simulink model "driveController"  (R2026a)
settings: Solver=FixedStepAuto  StopTime=20  FixedStep=0.001
StartFcn:
  | run("setupParams.m")
values from neighbouring files (symbols this model uses):
  aero_bal_r = 0.5    [setupParams.m]    (also in setupParamsSingle.m)
  Af = 1.1    [setupParams.m]    (also in setupParamsSingle.m)
  ay_limit = 15.0    (= 15)    [setupParams.m]    (also in setupParamsSingle.m)
  Cl = 1.0    (= 1)    [setupParams.m]    (also in setupParamsSingle.m)
  deathzone_APP = 5    [setupParams.m]    (also in setupParamsSingle.m)
  e_yaw_deadzone = 0.03    [setupParams.m]
  falling_slew_rate_torque = -500    [setupParams.m]    (also in setupParamsSingle.m)
  g = 9.81    [setupParams.m]    (also in setupParamsSingle.m)
  h_o = 0.35    [setupParams.m]    (also in setupParamsSingle.m)
  I_charge_max = 21    [setupParams.m]
  I_discharge_max = 90    [setupParams.m]
  K_roll_rear = 0.6    [setupParams.m]    (also in setupParamsSingle.m = 0.5)
  Kus = 0.03    [setupParams.m]    (also in setupParamsSingle.m = 0)
  l_f = 0.775    [setupParams.m]    (also in setupParamsSingle.m)
  launch_ramp_rate = 1000.0    (= 1000)    [setupParams.m]    (also in setupParamsSingle.m)
  launch_V_thresh = 5.0    (= 5)    [setupParams.m]    (also in setupParamsSingle.m)
  mass = 320    [setupParams.m]    (also in setupParamsSingle.m = 300)
  mu = 1.5    [setupParams.m]    (also in setupParamsSingle.m)
  nominal_ramp_rate = 1000.0    (= 1000)    [setupParams.m]    (also in setupParamsSingle.m)
  overslip_factor = 1.01    [setupParams.m]    (also in setupParamsSingle.m = 1.13)
  pedal_bp = (0:10:100)'    [setupParams.m]    (also in setupParamsSingle.m)
  pedal_map = (pedal_bp / 100) .^ pedal_alpha    [setupParams.m]    (also in setupParamsSingle.m = (pedal_bp / 100) .^ pedal_alpha.Value)
  R_wheel = 0.2032    [setupParams.m]    (also in setupParamsSingle.m)
  regen_I_cont_A = 14.0    (= 14)    [setupParams.m]    (also in setupParamsSingle.m)
  regen_I_peak_A = 21.0    (= 21)    [setupParams.m]    (also in setupParamsSingle.m)
  regen_I_peak_dur_s = 4.0    (= 4)    [setupParams.m]    (also in setupParamsSingle.m)
  regen_P_batt_max_W = 35000    [setupParams.m]    (also in setupParamsSingle.m)
  regen_pedal_thr = 5.0    (= 5)    [setupParams.m]    (also in setupParamsSingle.m = 10)
  regen_speed_crit_rpm = 1000    [setupParams.m]    (also in setupParamsSingle.m = 500)
  regen_speed_min_rpm = 4000    [setupParams.m]    (also in setupParamsSingle.m = 3000)
  regen_T_max = 9    [setupParams.m]    (also in setupParamsSingle.m = Simulink.Parameter(T_rated.Value/2))
  rho = 1.225    [setupParams.m]    (also in setupParamsSingle.m)
  rid_eff = 0.80    (= 0.8)    [setupParams.m]    (also in setupParamsSingle.m)
  rid_ratio = 15    [setupParams.m]    (also in setupParamsSingle.m)
  rising_slew_rate_torque = 100    [setupParams.m]    (also in setupParamsSingle.m)
  rpm_safe_threshold = 100    [setupParams.m]
  slip_bc_coeff = 10    [setupParams.m]    (also in setupParamsSingle.m = Simulink.Parameter(1.5))
  slip_filt_N = 80    [setupParams.m]    (also in setupParamsSingle.m = 15)
  slip_Kd = 0.8    [setupParams.m]    (also in setupParamsSingle.m = Simulink.Parameter(5.0))
  slip_Ki = 13.0    (= 13)    [setupParams.m]    (also in setupParamsSingle.m = Simulink.Parameter(110.0))
  slip_Kp = 50.0    (= 50)    [setupParams.m]    (also in setupParamsSingle.m = Simulink.Parameter(180.0))
  slip_low_sat = 0.0    (= 0)    [setupParams.m]    (also in setupParamsSingle.m)
  slip_up_sat = 25    [setupParams.m]    (also in setupParamsSingle.m = 21)
  slip_V_min = 3    [setupParams.m]    (also in setupParamsSingle.m = 1)
  steer_ratio = 4.2    [pure_pursuit.m]    (also in setupParams.m; setupParamsSingle.m)
  steering_deadband = 1    [setupParams.m]
  T_headroom_k = 13.0    (= 13)    [setupParams.m]    (also in setupParamsSingle.m = Simulink.Parameter(5.0))
  T_headroom_max = 9    [setupParams.m]    (also in setupParamsSingle.m = Simulink.Parameter(5.0))
  T_peak = 20    [setupParams.m]    (also in setupParamsSingle.m = 21)
  T_rated = 9.8    [setupParams.m]    (also in setupParamsSingle.m = Simulink.Parameter(9.8))
  track_width = (track_width_r + track_width_f)/2    (= 1.2)    [setupParams.m]    (also in setupParamsSingle.m = sqrt(track_width_r^2 + track_width_f^2))
  track_width_r = 1.2    [setupParams.m]    (also in setupParamsSingle.m)
  Ts = 0.01    [setupParams.m]    (also in setupParamsSingle.m)
  tvc_bc = 17    [setupParams.m]
  tvc_D_thresh = 0.060    (= 0.06)    [setupParams.m]    (also in setupParamsSingle.m)
  tvc_D_thresh_off = 0.03    [setupParams.m]    (also in setupParamsSingle.m)
  tvc_Kd = 100    [setupParams.m]    (also in setupParamsSingle.m = Simulink.Parameter(5))
  tvc_Ki = 150    [setupParams.m]    (also in setupParamsSingle.m = Simulink.Parameter(10))
  tvc_Kp = 650    [setupParams.m]    (also in setupParamsSingle.m = Simulink.Parameter(70))
  tvc_N_filter = 25    [setupParams.m]    (also in setupParamsSingle.m = Simulink.Parameter(20))
  tvc_sat_dMz = 700    [setupParams.m]    (also in setupParamsSingle.m = Simulink.Parameter(10.0))
  tvc_throttle_on = 3.0    (= 3)    [setupParams.m]    (also in setupParamsSingle.m = Simulink.Parameter(3.0))
  tvc_tr = 5    [setupParams.m]    (also in setupParamsSingle.m = Simulink.Parameter(1.0))
  tvc_V_off = 2.0    (= 2)    [setupParams.m]    (also in setupParamsSingle.m = Simulink.Parameter(2.0))
  tvc_V_on = 4.0    (= 4)    [setupParams.m]    (also in setupParamsSingle.m = Simulink.Parameter(4.0))
  tvc_yaw_thresh = 0.08    [setupParams.m]    (also in setupParamsSingle.m)
  tvc_yaw_thresh_off = 0.04    [setupParams.m]    (also in setupParamsSingle.m)
  V_dc = 540    [setupParams.m]    (also in setupParamsSingle.m)
  V_dc_p = Simulink.Parameter(V_dc)    [setupParams.m]
  wheelbase = l_f + l_r    (= 1.55)    [setupParams.m]    (also in setupParamsSingle.m)
libraries: simulink x5, slpidlib x3
settings Model: Creator=Utente  LastModifiedBy=Utente
settings SolverCC: EnableFixedStepZeroCrossing=on
settings HardwareCC: ProdLargestAtomicInteger=Long  ProdLargestAtomicFloat=Double  ProdHWDeviceType=ARM Compatible->ARM Cortex-M
settings RTWCC: SystemTargetFile=ert.tlc  GenCodeOnly=on  Toolchain=GNU Tools for STM32  DataTypeReplacement=CDataTypesFixedWidth  Description=Embedded Coder
settings ERTTargetCC: MaxIdInt64=INT64_MAX  MinIdInt64=INT64_MIN  MaxIdUint64=UINT64_MAX  MaxIdInt32=INT32_MAX  MinIdInt32=INT32_MIN  MaxIdUint32=UINT32_MAX  MaxIdInt16=INT16_MAX  MinIdInt16=INT16_MIN  MaxIdUint16=UINT16_MAX  MaxIdInt8=INT8_MAX  MinIdInt8=INT8_MIN  MaxIdUint8=UINT8_MAX  GenerateSampleERTMain=on

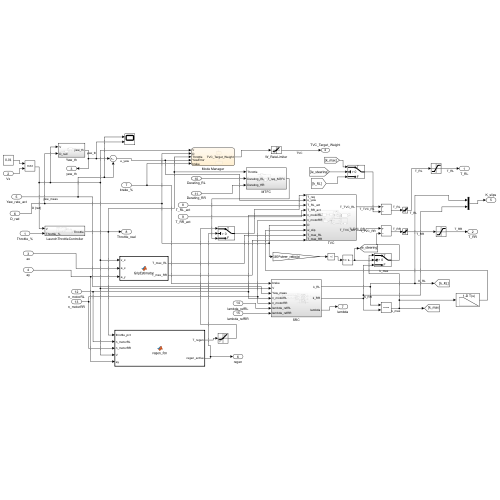
[thumbnail: Simulink's stored preview of the top-level diagram]
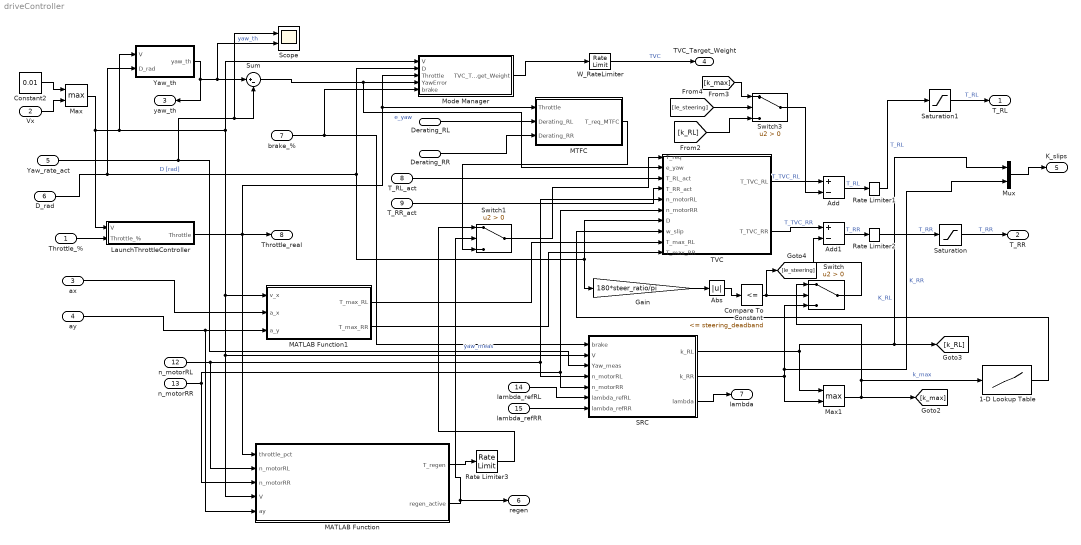
== system driveController ==
  Throttle_% : Inport
  Vx : Inport  Port=2
  ax : Inport  Port=3
  ay : Inport  Port=4
  Yaw_rate_act : Inport  Port=5
  D_rad : Inport  Port=6
  brake_% : Inport  Port=7
  T_RL_act : Inport  Port=8
  T_RR_act : Inport  Port=9
  Derating_RL : Inport  Port=10
  Derating_RR : Inport  Port=11
  n_motorRL : Inport  Port=12
  n_motorRR : Inport  Port=13
  lambda_refRL : Inport  Port=14
  lambda_refRR : Inport  Port=15
  1-D Lookup Table : Lookup_n-D  NumberOfTableDimensions=1  BreakpointsForDimension1=[0,3,12]  Table=[1,1,0]  ExtrapMethod=Clip  UseLastTableValue=on  InternalRulePriority=Speed  RndMeth=Simplest
  Abs : Abs  SaturateOnIntegerOverflow=off
  Add : Sum  Inputs=+-
  Add1 : Sum  Inputs=+-
  Compare To Constant : simulink/Logic and Bit Operations/Compare To Constant  relop=<=  const=steering_deadband  OutDataTypeStr=boolean
  Constant2 : Constant  Value=0.01
  Gain : Gain  Gain=180*steer_ratio/pi
  LaunchThrottleController : Subsystem
  MATLAB Function : MATLAB Function  TreatAsAtomicUnit=on
  MATLAB Function1 : MATLAB Function  TreatAsAtomicUnit=on
  MTFC : Subsystem
  Max : MinMax  Function=max  Inputs=2
  Max1 : MinMax  Function=max  Inputs=2
  Mode Manager : Stateflow chart  TreatAsAtomicUnit=on
  Mux : Mux  Inputs=2
  Rate Limiter1 : RateLimiter  RisingSlewLimit=rising_slew_rate_torque  FallingSlewLimit=falling_slew_rate_torque  SampleTimeMode=inherited
  Rate Limiter2 : RateLimiter  RisingSlewLimit=rising_slew_rate_torque  FallingSlewLimit=falling_slew_rate_torque  SampleTimeMode=inherited
  Rate Limiter3 : RateLimiter  RisingSlewLimit=60  FallingSlewLimit=-20  SampleTimeMode=inherited
  SRC : Subsystem
  Saturation : Saturate  UpperLimit=T_peak  LowerLimit=-regen_T_max
  Saturation1 : Saturate  UpperLimit=T_peak  LowerLimit=-regen_T_max
  Scope : Scope  NumInputPorts=2
      settings: ActiveDisplayYMinimum=-1.2846466868170756  ActiveDisplayYMaximum=1.5088492229704735
  Sum : Sum  Inputs=|+-
  Switch : Switch  Criteria=u2 > Threshold  SaturateOnIntegerOverflow=off  InputSameDT=off
  Switch1 : Switch  Criteria=u2 > Threshold  SaturateOnIntegerOverflow=off  InputSameDT=off
  Switch3 : Switch  Criteria=u2 > Threshold  SaturateOnIntegerOverflow=off  InputSameDT=off
  TVC : Subsystem
  W_RateLimiter : RateLimiter  RisingSlewLimit=2  FallingSlewLimit=-2  SampleTimeMode=inherited
  Yaw_th : Subsystem
  T_RL : Outport
  T_RR : Outport  Port=2
  yaw_th : Outport  Port=3
  TVC_Target_Weight : Outport  Port=4
  K_slips : Outport  Port=5
  regen : Outport  Port=6
  lambda : Outport  Port=7
  Throttle_real : Outport  Port=8
  wires:
  [k_RL] -> Switch3/3
  Add/1 -> Rate Limiter1/1  "T_RL"
  Mode Manager/1(TVC_Target_Weight) -> W_RateLimiter/1
  n_motorRR/1 -> TVC/6(n_motorRR), SRC/5(n_motorRR), MATLAB Function/3(n_motorRR)
  SRC/1(k_RL) -> Mux/1, [k_RL], Max1/1  "K_RL"
  Max1/1 -> 1-D Lookup Table/1, Switch/1, [k_max]  "k_max"
  [le_steering] -> Switch3/2
  Saturation/1 -> T_RR/1  "T_RR"
  n_motorRL/1 -> TVC/5(n_motorRL), SRC/4(n_motorRL), MATLAB Function/2(n_motorRL)
  T_RL_act/1 -> TVC/3(T_RL_act)
  T_RR_act/1 -> TVC/4(T_RR_act)
  MATLAB Function1/1(T_max_RL) -> TVC/9(T_max_RL)
  lambda_refRL/1 -> SRC/6(lambda_refRL)
  MATLAB Function/1(T_regen) -> Rate Limiter3/1
  ay/1 -> MATLAB Function/5(ay), MATLAB Function1/3(a_y)
  Yaw_rate_act/1 -> SRC/3(Yaw_meas), Scope/1, Sum/2  "yaw_meas"
  Constant2/1 -> Max/1
  Rate Limiter3/1 -> Switch1/1
  D_rad/1 -> TVC/7(D), Gain/1, Mode Manager/2(D), Yaw_th/2(D_rad)  "D [rad]"
  Derating_RR/1 -> MTFC/3(Derating_RR)
  Switch3/1 -> Add/2
  Add1/1 -> Rate Limiter2/1  "T_RR"
  Mux/1 -> K_slips/1
  brake_%/1 -> SRC/1(brake), Mode Manager/5(brake)
  W_RateLimiter/1 -> TVC_Target_Weight/1  "TVC"
  ax/1 -> MATLAB Function1/2(a_x)
  lambda_refRR/1 -> SRC/7(lambda_refRR)
  MATLAB Function1/2(T_max_RR) -> TVC/10(T_max_RR)
  Max/1 -> LaunchThrottleController/1(V), MATLAB Function/4(V), SRC/2(V), MATLAB Function1/1(v_x), Mode Manager/1(V), Yaw_th/1(V)
  LaunchThrottleController/1(Throttle) -> MATLAB Function/1(throttle_pct), Mode Manager/3(Throttle), MTFC/1(Throttle), Throttle_real/1
  Saturation1/1 -> T_RL/1  "T_RL"
  Vx/1 -> Max/2
  Yaw_th/1(yaw_th) -> Scope/2, Sum/1, yaw_th/1  "yaw_th"
  [k_max] -> Switch3/1
  MTFC/1(T_req_MTFC) -> Switch1/3
  TVC/1(T_TVC_RL) -> Add/1  "T_TVC_RL"
  Switch/1 -> Add1/2
  Compare To Constant/1 -> [le_steering], Switch/2
  MATLAB Function/2(regen_active) -> Switch1/2, regen/1
  1-D Lookup Table/1 -> TVC/8(w_slip)
  Switch1/1 -> TVC/1(T_req)
  TVC/2(T_TVC_RR) -> Add1/1  "T_TVC_RR"
  Derating_RL/1 -> MTFC/2(Derating_RL)
  Gain/1 -> Abs/1
  Throttle_%/1 -> LaunchThrottleController/2(Throttle_%)
  Abs/1 -> Compare To Constant/1
  Sum/1 -> TVC/2(e_yaw), Mode Manager/4(YawError)  "e_yaw"
  SRC/3(lambda) -> lambda/1
  Rate Limiter2/1 -> Saturation/1  "T_RR"
  Rate Limiter1/1 -> Saturation1/1  "T_RL"
  SRC/2(k_RR) -> Switch/3, Mux/2, Max1/2  "K_RR"

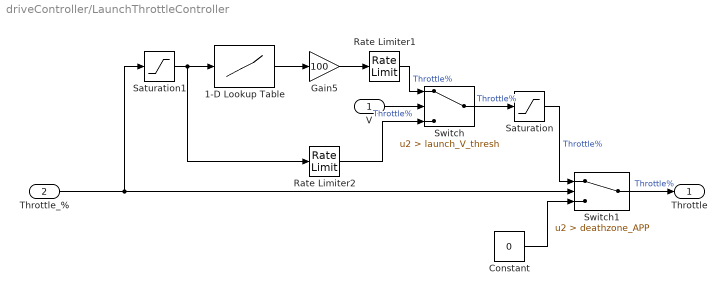
== system driveController/LaunchThrottleController ==
  V : Inport
  Throttle_% : Inport  Port=2
  1-D Lookup Table : Lookup_n-D  NumberOfTableDimensions=1  BreakpointsForDimension1=pedal_bp  Table=pedal_map  ExtrapMethod=Clip  UseLastTableValue=on  InternalRulePriority=Speed  RndMeth=Simplest
  Constant : Constant  Value=0
  Gain5 : Gain  Gain=100
  Rate Limiter1 : RateLimiter  RisingSlewLimit=launch_ramp_rate  FallingSlewLimit=-250  SampleTimeMode=inherited
  Rate Limiter2 : RateLimiter  RisingSlewLimit=nominal_ramp_rate  FallingSlewLimit=-250  SampleTimeMode=inherited
  Saturation : Saturate  UpperLimit=100  LowerLimit=0
  Saturation1 : Saturate  UpperLimit=100  LowerLimit=0
  Switch : Switch  Criteria=u2 > Threshold  Threshold=launch_V_thresh  SaturateOnIntegerOverflow=off  InputSameDT=off
  Switch1 : Switch  Criteria=u2 > Threshold  Threshold=deathzone_APP  SaturateOnIntegerOverflow=off  InputSameDT=off
  Throttle : Outport
  wires:
  1-D Lookup Table/1 -> Gain5/1
  Gain5/1 -> Rate Limiter1/1
  Switch1/1 -> Throttle/1  "Throttle%"
  Saturation1/1 -> Rate Limiter2/1, 1-D Lookup Table/1
  Rate Limiter2/1 -> Switch/3  "Throttle%"
  Rate Limiter1/1 -> Switch/1  "Throttle%"
  V/1 -> Switch/2
  Switch/1 -> Saturation/1  "Throttle%"
  Saturation/1 -> Switch1/1  "Throttle%"
  Constant/1 -> Switch1/3
  Throttle_%/1 -> Saturation1/1, Switch1/2

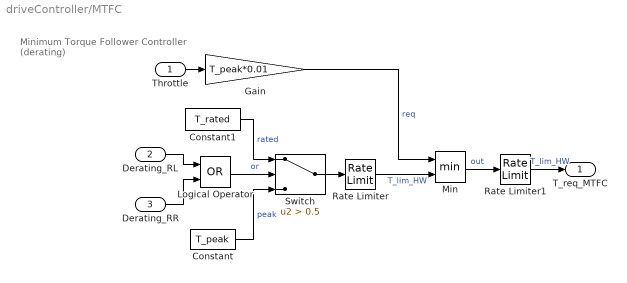
== system driveController/MTFC ==
  note: Minimum Torque Follower Controller
      | (derating)
  Throttle : Inport
  Derating_RL : Inport  Port=2
  Derating_RR : Inport  Port=3
  Constant : Constant  Value=T_peak
  Constant1 : Constant  Value=T_rated
  Gain : Gain  Gain=T_peak*0.01
  Logical Operator : Logic  Operator=OR  AllPortsSameDT=off  OutDataTypeStr=boolean
  Min : MinMax  Inputs=2
  Rate Limiter : RateLimiter  RisingSlewLimit=250  FallingSlewLimit=-250  SampleTimeMode=inherited
  Rate Limiter1 : RateLimiter  RisingSlewLimit=250  FallingSlewLimit=-10  SampleTimeMode=inherited
  Switch : Switch  Criteria=u2 > Threshold  Threshold=0.5  SaturateOnIntegerOverflow=off  InputSameDT=off
  T_req_MTFC : Outport
  wires:
  Min/1 -> Rate Limiter1/1  "out"
  Derating_RL/1 -> Logical Operator/1
  Logical Operator/1 -> Switch/2  "or"
  Derating_RR/1 -> Logical Operator/2
  Throttle/1 -> Gain/1
  Constant1/1 -> Switch/1  "rated"
  Constant/1 -> Switch/3  "peak"
  Switch/1 -> Rate Limiter/1
  Gain/1 -> Min/1  "req"
  Rate Limiter/1 -> Min/2  "T_lim_HW"
  Rate Limiter1/1 -> T_req_MTFC/1  "T_lim_HW"

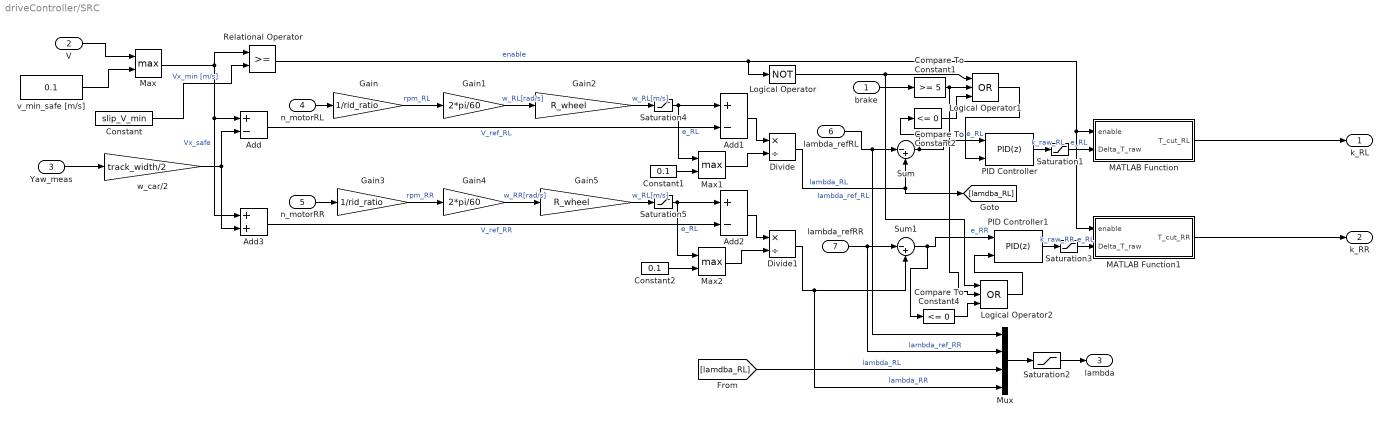
== system driveController/SRC ==
  brake : Inport
  V : Inport  Port=2
  Yaw_meas : Inport  Port=3
  n_motorRL : Inport  Port=4
  n_motorRR : Inport  Port=5
  lambda_refRL : Inport  Port=6
  lambda_refRR : Inport  Port=7
  Add : Sum  Inputs=+-
  Add1 : Sum  Inputs=+-
  Add2 : Sum  Inputs=+-
  Add3 : Sum
  Compare To Constant1 : simulink/Logic and Bit Operations/Compare To Constant  relop=>=  const=5  OutDataTypeStr=boolean
  Compare To Constant2 : simulink/Logic and Bit Operations/Compare To Constant  relop=<=  const=0  OutDataTypeStr=boolean
  Compare To Constant4 : simulink/Logic and Bit Operations/Compare To Constant  relop=<=  const=0  OutDataTypeStr=boolean
  Constant : Constant  Value=slip_V_min
  Constant1 : Constant  Value=0.1
  Constant2 : Constant  Value=0.1
  Divide : Product  Inputs=*/
  Divide1 : Product  Inputs=*/
  Gain : Gain  Gain=1/rid_ratio
  Gain1 : Gain  Gain=2*pi/60
  Gain2 : Gain  Gain=R_wheel
  Gain3 : Gain  Gain=1/rid_ratio
  Gain4 : Gain  Gain=2*pi/60
  Gain5 : Gain  Gain=R_wheel
  Logical Operator : Logic  Operator=NOT  AllPortsSameDT=off  OutDataTypeStr=boolean
  Logical Operator1 : Logic  Operator=OR  Inputs=3  AllPortsSameDT=off  OutDataTypeStr=boolean
  Logical Operator2 : Logic  Operator=OR  Inputs=3  AllPortsSameDT=off  OutDataTypeStr=boolean
  MATLAB Function : MATLAB Function  TreatAsAtomicUnit=on
  MATLAB Function1 : MATLAB Function  TreatAsAtomicUnit=on
  Max : MinMax  Function=max  Inputs=2
  Max1 : MinMax  Function=max  Inputs=2
  Max2 : MinMax  Function=max  Inputs=2
  Mux : Mux
  PID Controller : slpidlib/PID Controller  Controller=PID  Form=Parallel  TimeDomain=Discrete-time  UseExternalTs=off  SampleTime=Ts  IntegratorMethod=Forward Euler  FilterMethod=Forward Euler  ControllerParametersSource=internal  P=slip_Kp  I=slip_Ki  UseKiTs=off  D=slip_Kd  UseExternalDerivativeSource=off  N=slip_filt_N  UseFilter=on  TunerSelectOption=Transfer Function Based (PID Tuner App)  InitialConditionSource=internal  InitialConditionForIntegrator=0  InitialConditionForFilter=0  DifferentiatorICPrevScaledInput=0  ExternalReset=level  TrackingMode=off  Kt=1  LimitOutput=on  SatLimitsSource=internal  UpperSaturationLimit=slip_up_sat  LowerSaturationLimit=slip_low_sat  LinearizeAsGain=on  AntiWindupMode=back-calculation  Kb=slip_bc_coeff  LimitIntegrator=on  UpperIntegratorSaturationLimit=slip_up_sat  LowerIntegratorSaturationLimit=slip_low_sat  POutMin=[]  POutMax=[]  IOutMin=[]  IOutMax=[]  DOutMin=[]  DOutMax=[]  NOutMin=[]  NOutMax=[]  SumOutMin=[]  SumOutMax=[]  SaturationOutMin=[]  SaturationOutMax=[]  PParamMin=[]  PParamMax=[]  IParamMin=[]  IParamMax=[]  DParamMin=[]  DParamMax=[]  NParamMin=[]  NParamMax=[]  KbParamMin=[]  KbParamMax=[]  KtParamMin=[]  KtParamMax=[]  KbOutMin=[]  KbOutMax=[]  KtOutMin=[]  KtOutMax=[]  IntegratorOutMin=[]  IntegratorOutMax=[]  FilterOutMin=[]  FilterOutMax=[]  SumI1OutMin=[]  SumI1OutMax=[]  SumI2OutMin=[]  SumI2OutMax=[]  SumI3OutMin=[]  SumI3OutMax=[]  SumI4OutMin=[]  SumI4OutMax=[]  SumDOutMin=[]  SumDOutMax=[]  DifferentiatorOutMin=[]  DifferentiatorOutMax=[]  FilterDiffOutCoefMin=[]  FilterDiffOutCoefMax=[]  ReciprocalOutMin=[]  ReciprocalOutMax=[]  SumDenOutMin=[]  SumDenOutMax=[]  SumNumOutMin=[]  SumNumOutMax=[]  DivideOutMin=[]  DivideOutMax=[]  UdiffTsProdOutMin=[]  UdiffTsProdOutMax=[]  NTsProdOutMin=[]  NTsProdOutMax=[]  UintegralTsProdOutMin=[]  UintegralTsProdOutMax=[]  UngainTsProdOutMin=[]  UngainTsProdOutMax=[]  ClampingZeroOutDataTypeStr=Inherit: Inherit via back propagation  ClampingZeroOutMin=[]  ClampingZeroOutMax=[]  FilterDenConstantOutDataTypeStr=Inherit: Inherit via back propagation  FilterDenConstantOutMin=[]  FilterDenConstantOutMax=[]  PCopyOutDataTypeStr=Inherit: Inherit via back propagation  PCopyOutMin=[]  PCopyOutMax=[]  NCopyOutDataTypeStr=Inherit: Inherit via back propagation  NCopyOutMin=[]  NCopyOutMax=[]  IntegratorContinuousStateAttributes=''  IntegratorStateMustResolveToSignalObject=off  IntegratorRTWStateStorageClass=Auto  FilterContinuousStateAttributes=''  FilterStateMustResolveToSignalObject=off  FilterRTWStateStorageClass=Auto  ParallelPVariant=InternalParameters  IdealPVariant=Disabled  IVariant=InternalParameters  DVariant=InternalParameters  IntegratorVariant=Discrete  SatVariant=Enabled  AWVariant=BackCalculation  PCopyVariant=Disabled  TRVariant=Disabled  FdbkBlocksVariant=Forward  IdealPFdbkVariant=Disabled  SatFdbkVariant=Disabled  DerivativeFilterVariant=ForwardEulerFilter  NVariant=InternalParameters  NCopyVariant=Disabled  FilterICVariant=InternalICsFilter  IntegratorICVariant=InternalICs  ExternalResetVariant=ExternalReset  TRSumVariant=Passthrough  SumFdbkVariant=Disabled  SumVariant=Sum_PID  TsampFilterVariant=InternalTs  TsampNgainVariant=Passthrough  TsampIntegralVariant=Disabled_SignalSpec  ExternalSaturationOutDataTypeStr=Inherit: Same as second input  DerivativeSourceVariant=ErrorSignal  PreIntVariant=InternalPreInt
  PID Controller1 : slpidlib/PID Controller  Controller=PID  Form=Parallel  TimeDomain=Discrete-time  UseExternalTs=off  SampleTime=Ts  IntegratorMethod=Forward Euler  FilterMethod=Forward Euler  ControllerParametersSource=internal  P=slip_Kp  I=slip_Ki  UseKiTs=off  D=slip_Kd  UseExternalDerivativeSource=off  N=slip_filt_N  UseFilter=on  TunerSelectOption=Transfer Function Based (PID Tuner App)  InitialConditionSource=internal  InitialConditionForIntegrator=0  InitialConditionForFilter=0  DifferentiatorICPrevScaledInput=0  ExternalReset=level  TrackingMode=off  Kt=1  LimitOutput=on  SatLimitsSource=internal  UpperSaturationLimit=slip_up_sat  LowerSaturationLimit=slip_low_sat  LinearizeAsGain=on  AntiWindupMode=back-calculation  Kb=slip_bc_coeff  LimitIntegrator=on  UpperIntegratorSaturationLimit=slip_up_sat  LowerIntegratorSaturationLimit=slip_low_sat  POutMin=[]  POutMax=[]  IOutMin=[]  IOutMax=[]  DOutMin=[]  DOutMax=[]  NOutMin=[]  NOutMax=[]  SumOutMin=[]  SumOutMax=[]  SaturationOutMin=[]  SaturationOutMax=[]  PParamMin=[]  PParamMax=[]  IParamMin=[]  IParamMax=[]  DParamMin=[]  DParamMax=[]  NParamMin=[]  NParamMax=[]  KbParamMin=[]  KbParamMax=[]  KtParamMin=[]  KtParamMax=[]  KbOutMin=[]  KbOutMax=[]  KtOutMin=[]  KtOutMax=[]  IntegratorOutMin=[]  IntegratorOutMax=[]  FilterOutMin=[]  FilterOutMax=[]  SumI1OutMin=[]  SumI1OutMax=[]  SumI2OutMin=[]  SumI2OutMax=[]  SumI3OutMin=[]  SumI3OutMax=[]  SumI4OutMin=[]  SumI4OutMax=[]  SumDOutMin=[]  SumDOutMax=[]  DifferentiatorOutMin=[]  DifferentiatorOutMax=[]  FilterDiffOutCoefMin=[]  FilterDiffOutCoefMax=[]  ReciprocalOutMin=[]  ReciprocalOutMax=[]  SumDenOutMin=[]  SumDenOutMax=[]  SumNumOutMin=[]  SumNumOutMax=[]  DivideOutMin=[]  DivideOutMax=[]  UdiffTsProdOutMin=[]  UdiffTsProdOutMax=[]  NTsProdOutMin=[]  NTsProdOutMax=[]  UintegralTsProdOutMin=[]  UintegralTsProdOutMax=[]  UngainTsProdOutMin=[]  UngainTsProdOutMax=[]  ClampingZeroOutDataTypeStr=Inherit: Inherit via back propagation  ClampingZeroOutMin=[]  ClampingZeroOutMax=[]  FilterDenConstantOutDataTypeStr=Inherit: Inherit via back propagation  FilterDenConstantOutMin=[]  FilterDenConstantOutMax=[]  PCopyOutDataTypeStr=Inherit: Inherit via back propagation  PCopyOutMin=[]  PCopyOutMax=[]  NCopyOutDataTypeStr=Inherit: Inherit via back propagation  NCopyOutMin=[]  NCopyOutMax=[]  IntegratorContinuousStateAttributes=''  IntegratorStateMustResolveToSignalObject=off  IntegratorRTWStateStorageClass=Auto  FilterContinuousStateAttributes=''  FilterStateMustResolveToSignalObject=off  FilterRTWStateStorageClass=Auto  ParallelPVariant=InternalParameters  IdealPVariant=Disabled  IVariant=InternalParameters  DVariant=InternalParameters  IntegratorVariant=Discrete  SatVariant=Enabled  AWVariant=BackCalculation  PCopyVariant=Disabled  TRVariant=Disabled  FdbkBlocksVariant=Forward  IdealPFdbkVariant=Disabled  SatFdbkVariant=Disabled  DerivativeFilterVariant=ForwardEulerFilter  NVariant=InternalParameters  NCopyVariant=Disabled  FilterICVariant=InternalICsFilter  IntegratorICVariant=InternalICs  ExternalResetVariant=ExternalReset  TRSumVariant=Passthrough  SumFdbkVariant=Disabled  SumVariant=Sum_PID  TsampFilterVariant=InternalTs  TsampNgainVariant=Passthrough  TsampIntegralVariant=Disabled_SignalSpec  ExternalSaturationOutDataTypeStr=Inherit: Same as second input  DerivativeSourceVariant=ErrorSignal  PreIntVariant=InternalPreInt
  Relational Operator : RelationalOperator  OutDataTypeStr=boolean  RndMeth=Simplest  InputSameDT=off
  Saturation1 : Saturate  UpperLimit=inf  LowerLimit=-2
  Saturation2 : Saturate  UpperLimit=1  LowerLimit=0
  Saturation3 : Saturate  UpperLimit=inf  LowerLimit=-2
  Saturation4 : Saturate  UpperLimit=inf  LowerLimit=0
  Saturation5 : Saturate  UpperLimit=inf  LowerLimit=0
  Sum : Sum  Inputs=|-+
  Sum1 : Sum  Inputs=|-+
  v_min_safe [m/s] : Constant  Value=0.1
  w_car/2 : Gain  Gain=track_width/2
  k_RL : Outport
  k_RR : Outport  Port=2
  lambda : Outport  Port=3
  wires:
  V/1 -> Max/1
  v_min_safe [m/s]/1 -> Max/2
  Max/1 -> Relational Operator/1, Add3/1, Add/1  "Vx_safe"
  Constant/1 -> Relational Operator/2  "Vx_min [m/s]"
  Yaw_meas/1 -> w_car/2/1
  Add/1 -> Add1/2  "V_ref_RL"
  n_motorRL/1 -> Gain/1
  Gain/1 -> Gain1/1  "rpm_RL"
  Add1/1 -> Divide/1
  Divide/1 -> [lamdba_RL], Sum/2  "lambda_RL"
  w_car/2/1 -> Add3/2, Add/2
  Gain1/1 -> Gain2/1  "w_RL[rad/s]"
  Gain2/1 -> Saturation4/1  "w_RL[m/s]"
  Gain4/1 -> Gain5/1  "w_RR[rad/s]"
  Gain3/1 -> Gain4/1  "rpm_RR"
  Divide1/1 -> Sum1/2, Mux/4  "lambda_RR"
  n_motorRR/1 -> Gain3/1
  Add3/1 -> Add2/2  "V_ref_RR"
  Add2/1 -> Divide1/1
  Relational Operator/1 -> MATLAB Function1/1(enable), MATLAB Function/1(enable), Logical Operator/1  "enable"
  PID Controller/1 -> Saturation1/1  "k_raw_RL"
  MATLAB Function/1(T_cut_RL) -> k_RL/1
  PID Controller1/1 -> Saturation3/1  "k_raw_RR"
  lambda_refRR/1 -> Mux/2, Sum1/1  "lambda_ref_RR"
  MATLAB Function1/1(T_cut_RR) -> k_RR/1
  Sum1/1 -> Compare To Constant4/1, PID Controller1/1  "e_RR"
  Sum/1 -> PID Controller/1, Compare To Constant2/1  "e_RL"
  Max1/1 -> Divide/2
  Constant1/1 -> Max1/2
  Max2/1 -> Divide1/2
  Constant2/1 -> Max2/2
  Gain5/1 -> Saturation5/1  "w_RL[m/s]"
  Mux/1 -> Saturation2/1
  Saturation2/1 -> lambda/1
  Saturation1/1 -> MATLAB Function/2(Delta_T_raw)  "e_RL"
  Saturation3/1 -> MATLAB Function1/2(Delta_T_raw)  "e_RL"
  Logical Operator1/1 -> PID Controller/2
  [lamdba_RL] -> Mux/3  "lambda_RL"
  Saturation4/1 -> Max1/1, Add1/1  "e_RL"
  Saturation5/1 -> Max2/1, Add2/1  "e_RL"
  Logical Operator/1 -> Logical Operator2/1, Logical Operator1/1
  Compare To Constant2/1 -> Logical Operator1/3
  Compare To Constant4/1 -> Logical Operator2/3
  lambda_refRL/1 -> Mux/1, Sum/1  "lambda_ref_RL"
  Logical Operator2/1 -> PID Controller1/2
  brake/1 -> Compare To Constant1/1
  Compare To Constant1/1 -> Logical Operator2/2, Logical Operator1/2

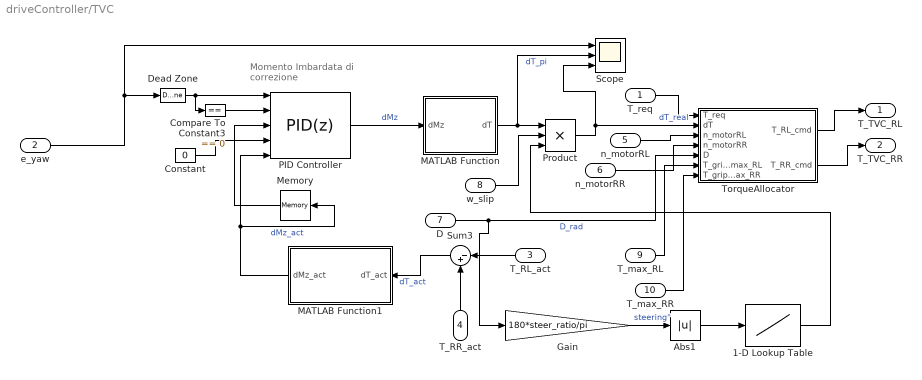
== system driveController/TVC ==
  note: Momento Imbardata di correzione
  T_req : Inport
  e_yaw : Inport  Port=2
  T_RL_act : Inport  Port=3
  T_RR_act : Inport  Port=4
  n_motorRL : Inport  Port=5
  n_motorRR : Inport  Port=6
  D : Inport  Port=7
  w_slip : Inport  Port=8
  T_max_RL : Inport  Port=9
  T_max_RR : Inport  Port=10
  1-D Lookup Table : Lookup_n-D  NumberOfTableDimensions=1  BreakpointsForDimension1=[0,steering_deadband,5]  Table=[0,0,1]  ExtrapMethod=Clip  UseLastTableValue=on  InternalRulePriority=Speed  RndMeth=Simplest
  Abs1 : Abs  SaturateOnIntegerOverflow=off
  Compare To Constant3 : simulink/Logic and Bit Operations/Compare To Constant  relop===  const=0  OutDataTypeStr=boolean
  Constant : Constant  Value=0
  Dead Zone : DeadZone  LowerValue=-e_yaw_deadzone  UpperValue=e_yaw_deadzone
  Gain : Gain  Gain=180*steer_ratio/pi
  MATLAB Function : MATLAB Function  TreatAsAtomicUnit=on
  MATLAB Function1 : MATLAB Function  TreatAsAtomicUnit=on
  Memory : Memory
  PID Controller : slpidlib/PID Controller  Controller=PID  Form=Parallel  TimeDomain=Discrete-time  UseExternalTs=off  SampleTime=Ts  IntegratorMethod=Forward Euler  FilterMethod=Forward Euler  ControllerParametersSource=internal  P=tvc_Kp  I=tvc_Ki  UseKiTs=off  D=tvc_Kd  UseExternalDerivativeSource=off  N=tvc_N_filter  UseFilter=on  TunerSelectOption=Transfer Function Based (PID Tuner App)  InitialConditionSource=external  InitialConditionForIntegrator=0  InitialConditionForFilter=0  DifferentiatorICPrevScaledInput=0  ExternalReset=level  TrackingMode=on  Kt=tvc_tr  LimitOutput=on  SatLimitsSource=internal  UpperSaturationLimit=tvc_sat_dMz  LowerSaturationLimit=-tvc_sat_dMz  LinearizeAsGain=on  AntiWindupMode=back-calculation  Kb=tvc_bc  LimitIntegrator=off  UpperIntegratorSaturationLimit=inf  LowerIntegratorSaturationLimit=-inf  POutMin=[]  POutMax=[]  IOutMin=[]  IOutMax=[]  DOutMin=[]  DOutMax=[]  NOutMin=[]  NOutMax=[]  SumOutMin=[]  SumOutMax=[]  SaturationOutMin=[]  SaturationOutMax=[]  PParamMin=[]  PParamMax=[]  IParamMin=[]  IParamMax=[]  DParamMin=[]  DParamMax=[]  NParamMin=[]  NParamMax=[]  KbParamMin=[]  KbParamMax=[]  KtParamMin=[]  KtParamMax=[]  KbOutMin=[]  KbOutMax=[]  KtOutMin=[]  KtOutMax=[]  IntegratorOutMin=[]  IntegratorOutMax=[]  FilterOutMin=[]  FilterOutMax=[]  SumI1OutMin=[]  SumI1OutMax=[]  SumI2OutMin=[]  SumI2OutMax=[]  SumI3OutMin=[]  SumI3OutMax=[]  SumI4OutMin=[]  SumI4OutMax=[]  SumDOutMin=[]  SumDOutMax=[]  DifferentiatorOutMin=[]  DifferentiatorOutMax=[]  FilterDiffOutCoefMin=[]  FilterDiffOutCoefMax=[]  ReciprocalOutMin=[]  ReciprocalOutMax=[]  SumDenOutMin=[]  SumDenOutMax=[]  SumNumOutMin=[]  SumNumOutMax=[]  DivideOutMin=[]  DivideOutMax=[]  UdiffTsProdOutMin=[]  UdiffTsProdOutMax=[]  NTsProdOutMin=[]  NTsProdOutMax=[]  UintegralTsProdOutMin=[]  UintegralTsProdOutMax=[]  UngainTsProdOutMin=[]  UngainTsProdOutMax=[]  ClampingZeroOutDataTypeStr=Inherit: Inherit via back propagation  ClampingZeroOutMin=[]  ClampingZeroOutMax=[]  FilterDenConstantOutDataTypeStr=Inherit: Inherit via back propagation  FilterDenConstantOutMin=[]  FilterDenConstantOutMax=[]  PCopyOutDataTypeStr=Inherit: Inherit via back propagation  PCopyOutMin=[]  PCopyOutMax=[]  NCopyOutDataTypeStr=Inherit: Inherit via back propagation  NCopyOutMin=[]  NCopyOutMax=[]  IntegratorContinuousStateAttributes=''  IntegratorStateMustResolveToSignalObject=off  IntegratorRTWStateStorageClass=Auto  FilterContinuousStateAttributes=''  FilterStateMustResolveToSignalObject=off  FilterRTWStateStorageClass=Auto  ParallelPVariant=InternalParameters  IdealPVariant=Disabled  IVariant=InternalParameters  DVariant=InternalParameters  IntegratorVariant=Discrete  SatVariant=Enabled  AWVariant=BackCalculation  PCopyVariant=Disabled  TRVariant=Enabled  FdbkBlocksVariant=Forward  IdealPFdbkVariant=Disabled  SatFdbkVariant=Disabled  DerivativeFilterVariant=ForwardEulerFilter  NVariant=InternalParameters  NCopyVariant=Disabled  FilterICVariant=ExternalICs  IntegratorICVariant=ExternalICs  ExternalResetVariant=ExternalReset  TRSumVariant=TrackingMode  SumFdbkVariant=Disabled  SumVariant=Sum_PID  TsampFilterVariant=InternalTs  TsampNgainVariant=Passthrough  TsampIntegralVariant=Disabled_SignalSpec  ExternalSaturationOutDataTypeStr=Inherit: Same as second input  DerivativeSourceVariant=ErrorSignal  PreIntVariant=InternalPreInt
  Product : Product  Inputs=3
  Scope : Scope  NumInputPorts=3
      settings: ActiveDisplayYMinimum=-0.17006762266637193  ActiveDisplayYMaximum=0.69301535210007792
  Sum3 : Sum  Inputs=|-+
  TorqueAllocator : MATLAB Function  TreatAsAtomicUnit=on  SystemSampleTime=0.05
  T_TVC_RL : Outport
  T_TVC_RR : Outport  Port=2
  wires:
  PID Controller/1 -> MATLAB Function/1(dMz)  "dMz"
  Sum3/1 -> MATLAB Function1/1(dT_act)  "dT_act"
  MATLAB Function1/1(dMz_act) -> PID Controller/5, Memory/1  "dMz_act"
  T_RL_act/1 -> Sum3/1
  T_RR_act/1 -> Sum3/2
  Product/1 -> Scope/3, TorqueAllocator/2(dT)  "dT_real"
  TorqueAllocator/1(T_RL_cmd) -> T_TVC_RL/1
  TorqueAllocator/2(T_RR_cmd) -> T_TVC_RR/1
  n_motorRL/1 -> TorqueAllocator/3(n_motorRL)
  n_motorRR/1 -> TorqueAllocator/4(n_motorRR)
  Constant/1 -> PID Controller/4
  Memory/1 -> PID Controller/3
  e_yaw/1 -> Scope/1, Dead Zone/1
  D/1 -> TorqueAllocator/5(D), Gain/1  "D_rad"
  T_req/1 -> TorqueAllocator/1(T_req)
  Gain/1 -> Abs1/1  "steering°"
  MATLAB Function/1(dT) -> Scope/2, Product/1  "dT_pi"
  1-D Lookup Table/1 -> Product/3
  Abs1/1 -> 1-D Lookup Table/1
  w_slip/1 -> Product/2
  T_max_RL/1 -> TorqueAllocator/6(T_grip_max_RL)
  T_max_RR/1 -> TorqueAllocator/7(T_grip_max_RR)
  Dead Zone/1 -> Compare To Constant3/1, PID Controller/1
  Compare To Constant3/1 -> PID Controller/2

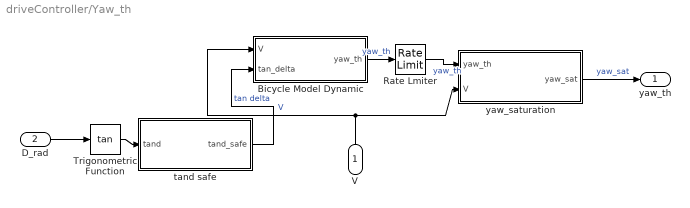
== system driveController/Yaw_th ==
  V : Inport
  D_rad : Inport  Port=2
  Bicycle Model Dynamic : MATLAB Function  TreatAsAtomicUnit=on
  Rate Lmiter : RateLimiter  SampleTimeMode=inherited
  Trigonometric Function : Trigonometry  Operator=tan
  tand safe : MATLAB Function  TreatAsAtomicUnit=on
  yaw_saturation : MATLAB Function  TreatAsAtomicUnit=on
  yaw_th : Outport
  wires:
  tand safe/1(tand_safe) -> Bicycle Model Dynamic/2(tan_delta)  "tan delta"
  Trigonometric Function/1 -> tand safe/1(tand)
  Bicycle Model Dynamic/1(yaw_th) -> Rate Lmiter/1  "yaw_th"
  V/1 -> Bicycle Model Dynamic/1(V), yaw_saturation/2(V)  "V"
  D_rad/1 -> Trigonometric Function/1
  Rate Lmiter/1 -> yaw_saturation/1(yaw_th)  "yaw_th"
  yaw_saturation/1(yaw_sat) -> yaw_th/1  "yaw_sat"

== matlab function driveController/SRC/MATLAB Function ==
  data: enable input; T_cut_RL output; Delta_T_raw input
function T_cut_RL = fcn(enable, Delta_T_raw)
    T_cut_RL = enable * Delta_T_raw;
end

== matlab function driveController/SRC/MATLAB Function1 ==
  data: enable input; T_cut_RR output; Delta_T_raw input
function T_cut_RR = fcn(enable, Delta_T_raw)
    T_cut_RR = enable * Delta_T_raw;
end

== matlab function driveController/TVC/MATLAB Function ==
  data: dMz input; dT output; R_wheel parameter; track_width parameter; rid_ratio parameter; rid_eff parameter
function dT = fcn(dMz, R_wheel, track_width, rid_ratio, rid_eff)
    dT = dMz * R_wheel / (track_width * rid_ratio * rid_eff);
end

== matlab function driveController/TVC/MATLAB Function1 ==
  data: dT_act input; dMz_act output; track_width parameter; R_wheel parameter; rid_ratio parameter; rid_eff parameter
function dMz_act = fcn(dT_act, track_width, R_wheel, rid_ratio, rid_eff)
    %Yaw moment (z) that the engines are currently delivering
    dMz_act = dT_act * track_width * rid_ratio * rid_eff / (2 * R_wheel);
end

== matlab function driveController/TVC/TorqueAllocator ==
  data: T_req input; T_RL_cmd output; dT input; n_motorRL input; n_motorRR input; T_RR_cmd output; D input; V_dc_p parameter; T_peak parameter; T_headroom_max parameter; T_headroom_k parameter; T_grip_max_RL input; T_grip_max_RR input; rpm_safe_threshold parameter; I_discharge_max parameter
function [T_RL_cmd, T_RR_cmd] = fcn(T_req, dT, n_motorRL, n_motorRR, D, ...
    V_dc_p, T_peak, T_headroom_max, T_headroom_k, T_grip_max_RL, T_grip_max_RR, rpm_safe_threshold, I_discharge_max)
    T_min = 0;
    
    % --- CALCOLO POTENZA MASSIMA (Inverter) ---
    P_max_inverter = V_dc_p * 58.33; 
    
    % --- CALCOLO LIMITI ELETTRICI (FIELD WEAKENING) ---
    w_RL = max(abs(n_motorRL) * (pi/30), 1.0); 
    w_RR = max(abs(n_motorRR) * (pi/30), 1.0);
    
    T_fw_L = P_max_inverter / w_RL;
    T_fw_R = P_max_inverter / w_RR;
    
    T_elec_max_RL = min(T_peak, T_fw_L);
    T_elec_max_RR = min(T_peak, T_fw_R);
    
    % --- LIMITI FISICI GLOBALI ---
    T_max_L = min(T_elec_max_RL, T_grip_max_RL);
    T_max_R = min(T_elec_max_RR, T_grip_max_RR);
    
    % ---  PROTEZIONE ASIMMETRIA E HEADROOM TVC ---
    T_lim_base = min(T_max_L, T_max_R);
    T_headroom = min(T_headroom_max, T_headroom_k * abs(D));
    
    T_lim_base_neg = -min(T_grip_max_RL, T_grip_max_RR); 
    
    if T_req >= 0
        T_req_eff = max(0, min(T_req, T_lim_base - T_headroom));
    else
        T_req_eff = max(T_lim_base_neg + T_headroom, min(0, T_req));
    end
    
    % ---  TEORICO TVC ---
    T_L = T_req_eff - dT;
    T_R = T_req_eff + dT;
    
    if (abs(n_motorRL) < rpm_safe_threshold) && (T_L < 0)
        T_L = 0;
    end
    if (abs(n_motorRR) < rpm_safe_threshold) && (T_R < 0)
        T_R = 0;
    end
    
    % --- LIMITAZIONE PROPORZIONALE POTENZA DC (DC Current Limit) ---
    P_req_L = max(0, T_L * w_RL);
    P_req_R = max(0, T_R * w_RR);
    P_tot_req = P_req_L + P_req_R;
    
    P_limit_dc = V_dc_p * I_discharge_max;
    
    if P_tot_req > P_limit_dc
        scale_factor = P_limit_dc / P_tot_req;
        T_L = T_L * scale_factor;
        T_R = T_R * scale_factor;
    end
    
    % --- SATURAZIONE FINALE ---
    T_RL_cmd = max(-T_grip_max_RL, min(T_max_L, T_L));
    T_RR_cmd = max(-T_grip_max_RR, min(T_max_R, T_R));
end

== matlab function driveController/Yaw_th/Bicycle Model Dynamic ==
  data: V input; yaw_th output; tan_delta input; wheelbase parameter; Kus parameter
function yaw_th = fcn(V,tan_delta,wheelbase,Kus)
% L = 1.55; %passo veicolo [m]
% yaw_th = (V / L) * tand;
%
  
yaw_th = (V / wheelbase) * tan_delta / (1 + Kus * V^2);



end

== matlab function driveController/Yaw_th/tand safe ==
  data: tand input; tand_safe output; angle_limit_d parameter
function tand_safe = fcn(tand,angle_limit_d)
    soglia = tan(angle_limit_d*pi/180);  % 2° rad
    
    if abs(tand) < soglia
        tand_safe = 0;  % 
    else
        tand_safe = tand;  
    end
end

== matlab function driveController/Yaw_th/yaw_saturation ==
  data: yaw_th input; yaw_sat output; V input; mu parameter; g parameter
function yaw_sat = fcn(yaw_th, V,mu, g)
    V_calc = max(V, 0.5);
    
    yaw_max_abs = (mu * g) / V_calc;
    yaw_sat = sign(yaw_th) * min(abs(yaw_th), yaw_max_abs);
end

== matlab function driveController/MATLAB Function ==
  settings: updateMethod=DISCRETE
  data: throttle_pct input; T_regen output; n_motorRL input; n_motorRR input; V input; regen_active output; Ts parameter; regen_T_max parameter; regen_pedal_thr parameter; regen_speed_min_rpm parameter; regen_speed_crit_rpm parameter; regen_I_peak_A parameter; regen_I_cont_A parameter; regen_I_peak_dur_s parameter; regen_P_batt_max_W parameter; V_dc parameter; ay input; ay_limit parameter; I_charge_max parameter
function [T_regen, regen_active] = regen_fcn( ...
        throttle_pct, n_motorRL, n_motorRR, V, Ts, ...
        regen_T_max, regen_pedal_thr, regen_speed_min_rpm, regen_speed_crit_rpm, ...
        regen_I_peak_A, regen_I_cont_A, regen_I_peak_dur_s, ...
        regen_P_batt_max_W, V_dc, ay, ay_limit, I_charge_max)

    persistent t_elapsed_s;
    if isempty(t_elapsed_s)
        t_elapsed_s = 0.0;
    end
    speed_avg_rpm = (abs(n_motorRL) + abs(n_motorRR)) * 0.5;
    
    % ---- condizione di abilitazione regen 
    should_regen = (throttle_pct <= regen_pedal_thr) && ...
                   (speed_avg_rpm > regen_speed_crit_rpm) && ...
                   (V > 0.5);
    if ~should_regen
        t_elapsed_s = 0.0;
        T_regen = 0;
        regen_active = 0.0;
        return;
    end
    
    t_elapsed_s = t_elapsed_s + Ts;
    
    % ---- Stage 1: coppia pedal-dipendente [Nm, negativa] ----------------
    pedal_norm = throttle_pct / regen_pedal_thr;
    T_s1 = -regen_T_max * (1.0 - pedal_norm);
    
    if n_motorRL < regen_speed_min_rpm || n_motorRR < regen_speed_min_rpm
        t_elapsed_s = 0.0;
        T_regen = 0;
        regen_active = 0.0;
        return;
    end
    % ---- Stage 2: fade-out velocità -------------------------------------
    if speed_avg_rpm >= regen_speed_min_rpm
        k_vel = 1.0;
    else
        k_vel = speed_avg_rpm / regen_speed_min_rpm;
    end
    T_s2 = T_s1 * k_vel;
    
    % ---- Stage 3: limite potenza batteria (per motore = totale/2) -------
    omega_rad_s = (2.0 * pi * speed_avg_rpm) / 60.0;
    omega_safe  = max(omega_rad_s, 1.0);          
    T_P_lim     = (regen_P_batt_max_W * 0.5) / omega_safe;
    T_s3        = max(T_s2, -T_P_lim);            
    
    % --- NUOVO: INCROCIO LIMITI DI CORRENTE BMS ---
    if t_elapsed_s < regen_I_peak_dur_s
        I_lim_teorico = regen_I_peak_A;    
    else
        I_lim_teorico = regen_I_cont_A;   
    end
    
    % Sceglie il limite più severo tra la logica timer e il CAN del BMS
    I_lim_effettivo = min(I_lim_teorico, I_charge_max);
    I_lim_per_mot = I_lim_effettivo * 0.5;
    
    T_I_lim = (I_lim_per_mot * V_dc) / omega_safe;
    T_final = max(T_s3, -T_I_lim);
    
    % ---- Stage 4: limite regen x curva ----------------------------------
    k_derating_ay = max(0.0, 1.0 - (abs(ay) / ay_limit));
    T_final = T_final * k_derating_ay;
    
    % ---- output simmetrico sui due motori -------------------------------
    T_regen  = T_final;
    regen_active = 1; 
end

== matlab function driveController/MATLAB Function1 ==
  data: T_max_RL output; v_x input; a_x input; a_y input; T_max_RR output; mass parameter; g parameter; wheelbase parameter; l_f parameter; track_width_r parameter; mu parameter; h_o parameter; R_wheel parameter; Af parameter; Cl parameter; aero_bal_r parameter; K_roll_rear parameter; rho parameter; rid_ratio parameter; rid_eff parameter; overslip_factor parameter
function [T_max_RL, T_max_RR] = GripEstimator(v_x, a_x, a_y, mass, g, wheelbase, l_f, track_width_r,mu,h_o, R_wheel,Af, Cl, aero_bal_r, K_roll_rear, rho, rid_ratio,rid_eff, overslip_factor)
    % ---------------------------------------------------------
    % 1. CARICO BASE (Statico + Aerodinamico)
    % ---------------------------------------------------------
    Fz_stat_rear = mass * g * (l_f / wheelbase);
    
    Fz_aero_rear = 0.5 * rho * Af * Cl * (v_x^2) * aero_bal_r;
    
    Fz_base_wheel = (Fz_stat_rear + Fz_aero_rear) / 2;

   
    % 2. TRASFERIMENTI DI CARICO
    % Longitudinale: se a_x > 0 (accelerazione), il peso si sposta dietro (+)
    delta_Fz_long = 0.5 * (mass * a_x * h_o / wheelbase);
    
    % Laterale: dipende dall'accelerazione laterale a_y.
    % Convenzione: a_y < 0 per curva a destra-> peso si sposta a sinistra.
    delta_Fz_lat = (mass * a_y * h_o / track_width_r) * K_roll_rear;

    % 3. FORZE NORMALI FINALI SULLE RUOTE (Fz)
    Fz_RL = Fz_base_wheel + delta_Fz_long + delta_Fz_lat;
    Fz_RR = Fz_base_wheel + delta_Fz_long - delta_Fz_lat;

    % Prevenzione valori negativi (se la ruota interna si alza da terra, Fz = 0)
    if Fz_RL < 0
        Fz_RL = 0;
    end
    if Fz_RR < 0
        Fz_RR = 0;
    end
    

    
    % 4. CALCOLO COPPIA MASSIMA AI MOTORI
    % T = (F * R) / (tau * eff)

    % Parametri Pacejka (dal file .tir)
    Fz0 = 1112.0;
    PDX1 = 1.00347;
    PDX2 = -0.99198;

    % Calcolo mu dinamico per lato sinistro
    dfz_RL = (Fz_RL - Fz0) / Fz0;
    mu_RL = PDX1 + (PDX2 * dfz_RL);
    
    % Saturazione di sicurezza (evita mu negativi o assurdi)
    if mu_RL < 0.5; mu_RL = 0.5; end

    % Calcolo mu dinamico per lato destro
    dfz_RR = (Fz_RR - Fz0) / Fz0;
    mu_RR = PDX1 + (PDX2 * dfz_RR);
    if mu_RR < 0.5; mu_RR = 0.5; end
    
   

    % % Calcolo coppia massima ai motori usando il mu corretto
    % T_max_RL = (Fz_RL * mu_RL * R_wheel) / (rid_ratio * rid_eff);
    % T_max_RR = (Fz_RR * mu_RR * R_wheel) / (rid_ratio * rid_eff);

    % Calcolo coppia massima ai motori
     %T_max_RL = ((Fz_RL * mu_RL * R_wheel) / (rid_ratio * rid_eff)) * overslip_factor;
     %T_max_RR = ((Fz_RR * mu_RR * R_wheel) / (rid_ratio * rid_eff)) * overslip_factor;

    T_max_RL = (Fz_RL * mu * R_wheel) / (rid_ratio * rid_eff)* overslip_factor;
    T_max_RR = (Fz_RR * mu * R_wheel) / (rid_ratio * rid_eff)* overslip_factor;
end

== stateflow chart driveController/Mode Manager ==
  state IDLE_
    entry:
    TVC_Target_Weight = 0;
  note: %[brake > 0 || (Throttle < tvc_throttle_on && V <= tvc_V_off)]
  state TVC_
    entry: TVC_Target_Weight = 1;
  (default) -> IDLE_
  TVC_ -> IDLE_ : [V <= tvc_V_off]
  IDLE_ -> TVC_ : [V > tvc_V_on]
  data: TVC_Target_Weight output; V input; D input; Throttle input; YawError input; brake input; tvc_D_thresh parameter; tvc_yaw_thresh parameter; tvc_yaw_thresh_off parameter; tvc_throttle_on parameter; tvc_V_on parameter; tvc_V_off parameter; tvc_D_thresh_off parameter
